simulink model "lab3_ss_nominal_real_sim"  (R2024b)
settings: Solver=FixedStepAuto  StartTime=0.0  StopTime=20  FixedStep=0.001  RelTol=1e-3
undefined symbols (not defined in the file or in its folder): degs2rpm, deltaSS, DiscIntNeverNeededParam, National_Instruments, nominal_K, nominal_Nu, nominal_Nx, PCI, rpm2rads, sens, step_amplitude, t0_value, t1_value, Ts, wcSS
libraries: sldrtlib x3, simulink x1
settings Model: SimulationMode=external  ExtModeTrigDuration=50001  ExtModeTrigDurationFloating=50001  Creator=perondavid  LastModifiedBy=fasoloandr
settings DataIOCC: LoggingToFile=on
settings OptimizationCC: ReuseModelBlockBuffer=off
settings HardwareCC: ProdBitPerLong=64  ProdHWDeviceType=Intel->x86-64 (Linux 64)
settings RTWCC: Description=Simulink Desktop Real-Time  SystemTargetFile=sldrt.tlc  TemplateMakefile=sldrt.tmf  RTWCompilerOptimization=on  GPUComputeCapability=3.5
settings CodeAppCC: MaxIdLength=95
settings SimulinkDesktopRealTimeCC: TargetLibSuffix=_sldrt.a  TargetPreCompLibLocation=C:\Program Files\MATLAB\R2024b\toolbox\sldrt\lib\win64  ParMdlRefBuildCompliant=on

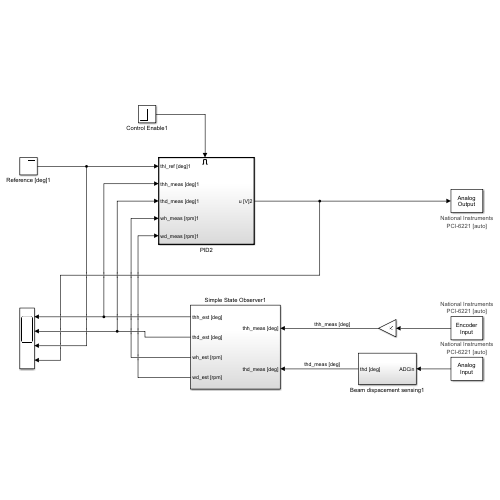
[thumbnail: Simulink's stored preview of the top-level diagram]
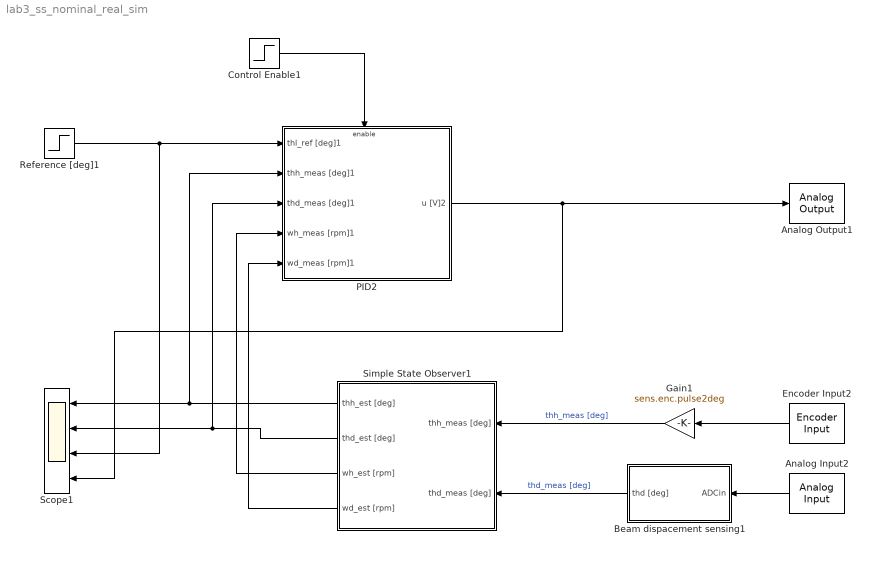
== system lab3_ss_nominal_real_sim ==
  Analog Input2 : sldrtlib/Analog Input  SampleTime=-1  MaxMissedTicks=10  ShowMissedTicks=off  YieldWhenWaiting=off  DrvName=National_Instruments/PCI-6221  DrvAddress=4294967295  DrvOptions=[0 0 0 2 0]  Channels=[3, 4]  RangeMode=1  VoltRange=2  DataType=1
      settings: AttributesFormatString=National Instruments\nPCI-6221 [auto]
  Analog Output1 : sldrtlib/Analog Output  SampleTime=-1  MaxMissedTicks=10  ShowMissedTicks=off  YieldWhenWaiting=off  DrvName=National_Instruments/PCI-6221  DrvAddress=4294967295  DrvOptions=[0 0 0 2 0]  Channels=1  RangeMode=1  VoltRange=1  InitialValue=0  FinalValue=0
      settings: AttributesFormatString=National Instruments\nPCI-6221 [auto]
  Beam dispacement sensing1 : Subsystem
  Control Enable1 : Step  Time=0.7  SampleTime=0
  Encoder Input2 : sldrtlib/Encoder Input  SampleTime=-1  MaxMissedTicks=10  ShowMissedTicks=off  YieldWhenWaiting=off  DrvName=National_Instruments/PCI-6221  DrvAddress=4294967295  DrvOptions=[0 0 0 2 0]  Channels=1  QuadMode=3  IndexPulse=1  InputFilter=Inf  DataType=1
      settings: AttributesFormatString=National Instruments\nPCI-6221 [auto]
  Gain1 : Gain  Gain=sens.enc.pulse2deg
  PID2 : Subsystem
  Reference [deg]1 : Step  Time=0  After=step_amplitude  SampleTime=Ts
  Scope1 : Scope  NumInputPorts=4
  Simple State Observer1 : Subsystem
  wires:
  Reference [deg]1/1 -> PID2/1(thl_ref [deg]1), Scope1/3
  Simple State Observer1/3(wh_est [rpm]) -> PID2/4(wh_meas [rpm]1)
  Simple State Observer1/4(wd_est [rpm]) -> PID2/5(wd_meas [rpm]1)
  Simple State Observer1/2(thd_est [deg]) -> PID2/3(thd_meas [deg]1), Scope1/2
  PID2/1(u [V]2) -> Analog Output1/1, Scope1/4
  Simple State Observer1/1(thh_est [deg]) -> PID2/2(thh_meas [deg]1), Scope1/1
  Beam dispacement sensing1/1(thd [deg]) -> Simple State Observer1/2(thd_meas [deg])  "thd_meas [deg]"
  Control Enable1/1 -> PID2/Enable
  Gain1/1 -> Simple State Observer1/1(thh_meas [deg])  "thh_meas [deg]"
  Encoder Input2/1 -> Gain1/1
  Analog Input2/1 -> Beam dispacement sensing1/1(ADCin)

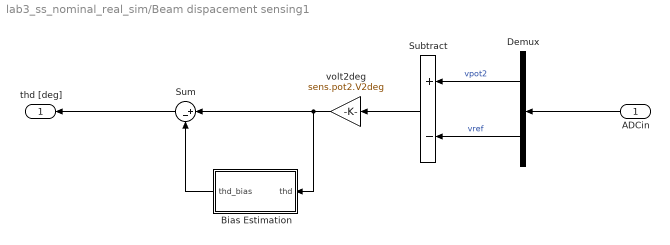
== system lab3_ss_nominal_real_sim/Beam dispacement sensing1 ==
  ADCin : Inport
  Bias Estimation : Subsystem
  Demux : Demux  Outputs=2
  Subtract : Sum  Inputs=+-
  Sum : Sum  Inputs=|+-
  volt2deg : Gain  Gain=sens.pot2.V2deg
  thd [deg] : Outport
  wires:
  Subtract/1 -> volt2deg/1
  volt2deg/1 -> Sum/1, Bias Estimation/1(thd)
  Sum/1 -> thd [deg]/1
  Bias Estimation/1(thd_bias) -> Sum/2
  ADCin/1 -> Demux/1
  Demux/1 -> Subtract/1  "vpot2"
  Demux/2 -> Subtract/2  "vref"

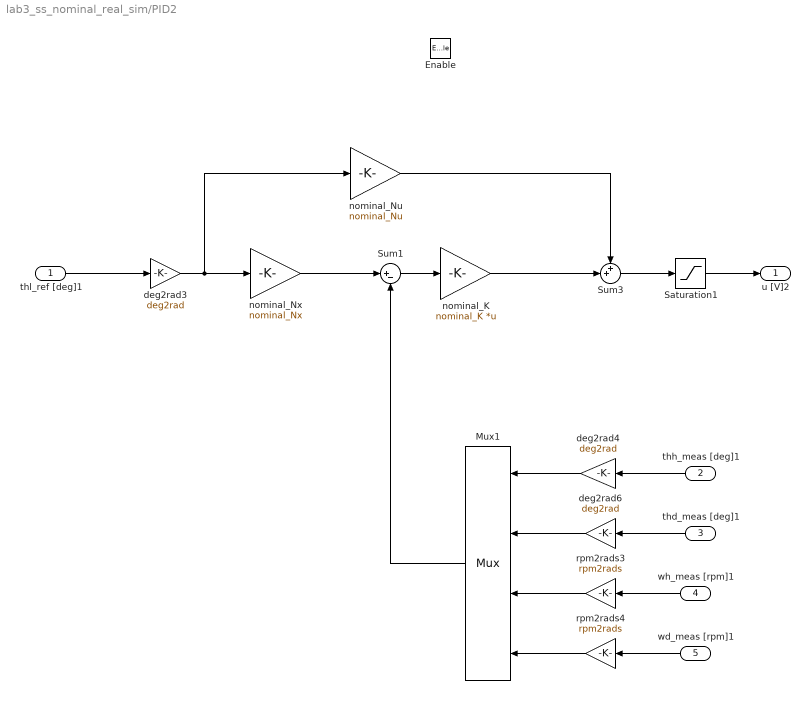
== system lab3_ss_nominal_real_sim/PID2 ==
  thl_ref [deg]1 : Inport
  thh_meas [deg]1 : Inport  Port=2
  thd_meas [deg]1 : Inport  Port=3
  wh_meas [rpm]1 : Inport  Port=4
  wd_meas [rpm]1 : Inport  Port=5
  Enable : EnablePort
  Mux1 : Mux
      settings: DisplayOption=signals
  Saturation1 : Saturate  UpperLimit=10  LowerLimit=-10
  Sum1 : Sum  Inputs=|+-
  Sum3 : Sum  Inputs=++|
  deg2rad3 : Gain  Gain=deg2rad
  deg2rad4 : Gain  Gain=deg2rad
  deg2rad6 : Gain  Gain=deg2rad
  nominal_K : Gain  Gain=nominal_K  Multiplication=Matrix(K*u)
  nominal_Nu : Gain  Gain=nominal_Nu
  nominal_Nx : Gain  Gain=nominal_Nx
  rpm2rads3 : Gain  Gain=rpm2rads
  rpm2rads4 : Gain  Gain=rpm2rads
  u [V]2 : Outport
  wires:
  deg2rad6/1 -> Mux1/2
  thh_meas [deg]1/1 -> deg2rad4/1
  nominal_Nx/1 -> Sum1/1
  Mux1/1 -> Sum1/2
  deg2rad4/1 -> Mux1/1
  rpm2rads4/1 -> Mux1/4
  Sum3/1 -> Saturation1/1
  thd_meas [deg]1/1 -> deg2rad6/1
  Sum1/1 -> nominal_K/1
  wh_meas [rpm]1/1 -> rpm2rads3/1
  nominal_K/1 -> Sum3/2
  rpm2rads3/1 -> Mux1/3
  deg2rad3/1 -> nominal_Nu/1, nominal_Nx/1
  nominal_Nu/1 -> Sum3/1
  wd_meas [rpm]1/1 -> rpm2rads4/1
  Saturation1/1 -> u [V]2/1
  thl_ref [deg]1/1 -> deg2rad3/1

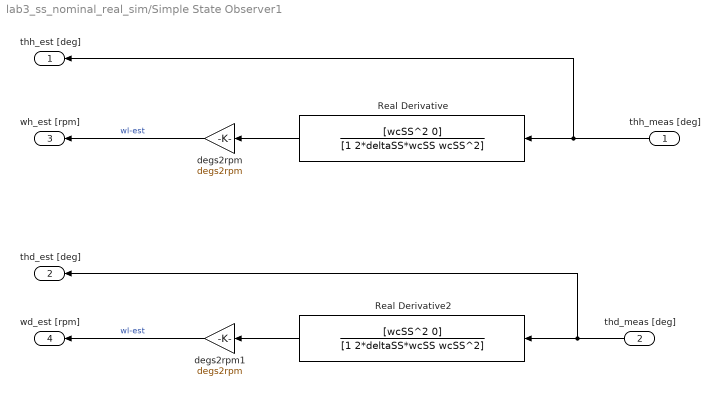
== system lab3_ss_nominal_real_sim/Simple State Observer1 ==
  thh_meas [deg] : Inport
  thd_meas [deg] : Inport  Port=2
  Real Derivative : TransferFcn  Numerator=[wcSS^2 0]  Denominator=[1 2*deltaSS*wcSS wcSS^2]
  Real Derivative2 : TransferFcn  Numerator=[wcSS^2 0]  Denominator=[1 2*deltaSS*wcSS wcSS^2]
  degs2rpm : Gain  Gain=degs2rpm
  degs2rpm1 : Gain  Gain=degs2rpm
  thh_est [deg] : Outport
  thd_est [deg] : Outport  Port=2
  wh_est [rpm] : Outport  Port=3
  wd_est [rpm] : Outport  Port=4
  wires:
  thd_meas [deg]/1 -> Real Derivative2/1, thd_est [deg]/1
  degs2rpm1/1 -> wd_est [rpm]/1  "wl-est"
  Real Derivative2/1 -> degs2rpm1/1
  degs2rpm/1 -> wh_est [rpm]/1  "wl-est"
  Real Derivative/1 -> degs2rpm/1
  thh_meas [deg]/1 -> thh_est [deg]/1, Real Derivative/1

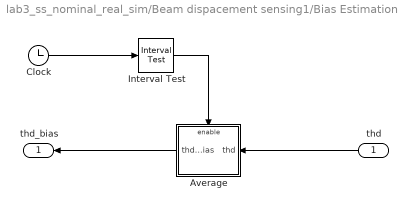
== system lab3_ss_nominal_real_sim/Beam dispacement sensing1/Bias Estimation ==
  thd : Inport
  Average : Subsystem
  Clock : Clock
  Interval Test : simulink/Logic and Bit Operations/Interval Test  IntervalClosedRight=on  uplimit=t1_value  IntervalClosedLeft=on  lowlimit=t0_value  OutDataTypeStr=boolean
  thd_bias : Outport
  wires:
  thd/1 -> Average/1(thd)
  Average/1(thd_bias) -> thd_bias/1
  Clock/1 -> Interval Test/1
  Interval Test/1 -> Average/Enable

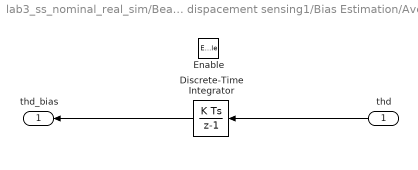
== system lab3_ss_nominal_real_sim/Beam dispacement sensing1/Bias Estimation/Average ==
  thd : Inport
  Enable : EnablePort
  Discrete-Time Integrator : DiscreteIntegrator  gainval=1/(t1_value-t0_value)  SampleTime=Ts  ICPrevOutput=DiscIntNeverNeededParam  ICPrevScaledInput=DiscIntNeverNeededParam
  thd_bias : Outport
  wires:
  thd/1 -> Discrete-Time Integrator/1
  Discrete-Time Integrator/1 -> thd_bias/1
